simulink model "SMA_Model_Controlled"  (R2021b)
settings: Solver=FixedStepAuto  StartTime=0.0  StopTime=100  FixedStep=1e-3  RelTol=1e-3  EnableMultiTasking=on
values from neighbouring files (symbols this model uses):
  c_heat = (530.21*delta_step + 446.67*delta_ramp)    (= 513.502)    [Model_Parameters.m]
  DerivativeGain = 13.5    [Model_Parameters.m]
  diameter = 5e-4    (= 0.0005)    [Model_Parameters.m]
  Ea = (75.896*delta_step + 80.942*delta_ramp)    (= 76.9052)    [Model_Parameters.m]
  Em = (45*delta_step + 45*delta_ramp)    (= 45)    [Model_Parameters.m]
  h = (39.765*delta_step + 28.06*delta_ramp)    (= 37.424)    [Model_Parameters.m]
  Initial_Rm = 1    [Model_Parameters.m]
  Initial_temperature = (25.147*delta_step + 26.734*delta_ramp)    (= 25.4644)    [Model_Parameters.m]
  IntegralGain = 0.275    [Model_Parameters.m]
  k1 = 0.0149669    [Model_Parameters.m]
  k2 = 0.001293    [Model_Parameters.m]
  L_init = 1.0    (= 1)    [Model_Parameters.m]
  lo = 1-0.0137    (= 0.9863)    [Model_Parameters.m]
  mu_minus = (52.26*delta_step + 52.208*delta_ramp)    (= 52.2496)    [Model_Parameters.m]
  mu_plus = (56.727*delta_step + 56.131*delta_ramp)    (= 56.6078)    [Model_Parameters.m]
  mVP = 0.020563    [Model_Parameters.m]
  PropotionalGain = 950    [Model_Parameters.m]
  qVP = -0.003866    [Model_Parameters.m]
  R = (3.1232*delta_step + 2.1253*delta_ramp)    (= 2.92362)    [Model_Parameters.m]
  rho = (5392.4*delta_step + 4835.5*delta_ramp)    (= 5281.02)    [Model_Parameters.m]
  sigma_minus = (8.711*delta_step + 8.5833*delta_ramp)    (= 8.68546)    [Model_Parameters.m]
  sigma_plus = (7.9951*delta_step + 8*delta_ramp)    (= 7.99608)    [Model_Parameters.m]
  Slider_Friction = (2.6643*delta_step + 0.84475*delta_ramp)    (= 2.30039)    [Model_Parameters.m]
  Slider_Mass = (0.020002*delta_step + 0.020016*delta_ramp)    (= 0.0200048)    [Model_Parameters.m]
  SupplyVoltage = (25.001*delta_step + 25.988*delta_ramp)    (= 25.1984)    [Model_Parameters.m]
  T_amb = (26.221*delta_step + 26.843*delta_ramp)    (= 26.3454)    [Model_Parameters.m]
libraries: fl_lib x7, simulink x5, ec_arm_cortex_a_lib x4, nesl_utility x4, dspsrcs4 x1
settings Model: ExtModeTrigDuration=1000000  Creator=barag  LastModifiedBy=barag
settings SolverCC: ZeroCrossAlgorithm=Adaptive  PositivePriorityOrder=on  AutoInsertRateTranBlk=on
settings OptimizationCC: EnhancedBackFolding=on  PassReuseOutputArgsAs=Individual arguments  ZeroExternalMemoryAtStartup=off  ZeroInternalMemoryAtStartup=off  MaxStackSize=64  OptimizeBlockOrder=speed  DifferentSizesBufferReuse=on  OptimizationCustomize=off  EfficientTunableParamExpr=on
settings DebuggingCC: MaskedZcDiagnostic=none  IgnoredZcDiagnostic=none  ParameterTunabilityLossMsg=error
settings HardwareCC: ProdBitPerPointer=32  ProdBitPerSizeT=32  ProdBitPerPtrDiffT=32  ProdLargestAtomicInteger=Long  ProdLargestAtomicFloat=Double  ProdWordSize=32  ProdHWDeviceType=ARM Compatible->ARM Cortex
settings SFSimCC: MATLABDynamicMemAlloc=off
settings RTWCC: Description=Embedded Coder  SystemTargetFile=ert.tlc  HardwareBoard=BeagleBone Black  TLCOptions="-aInlineSetEventsForThisBaseRateFcn=TLC_FALSE -aSuppressMultiTaskScheduler=TLC_FALSE  -aRateBasedStepFcn=0"  TemplateMakefile=ert_default_tmf  Toolchain=Linaro Toolchain v4.8
settings CodeAppCC: ForceParamTrailComments=on  IgnoreCustomStorageClasses=off  OperatorAnnotations=on  SimulinkDataObjDesc=on  SFDataObjDesc=on  InsertBlockDesc=on
settings ERTTargetCC: SupportContinuousTime=on

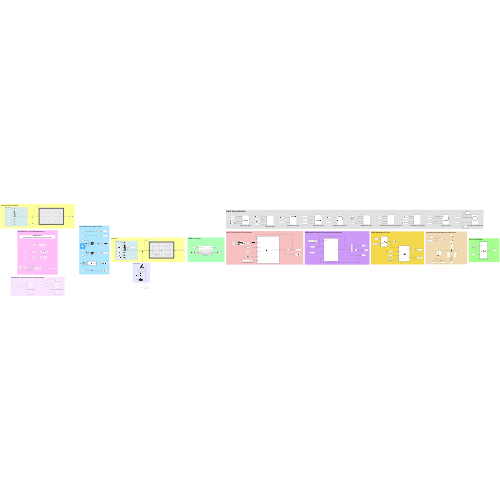
[thumbnail: Simulink's stored preview of the top-level diagram]
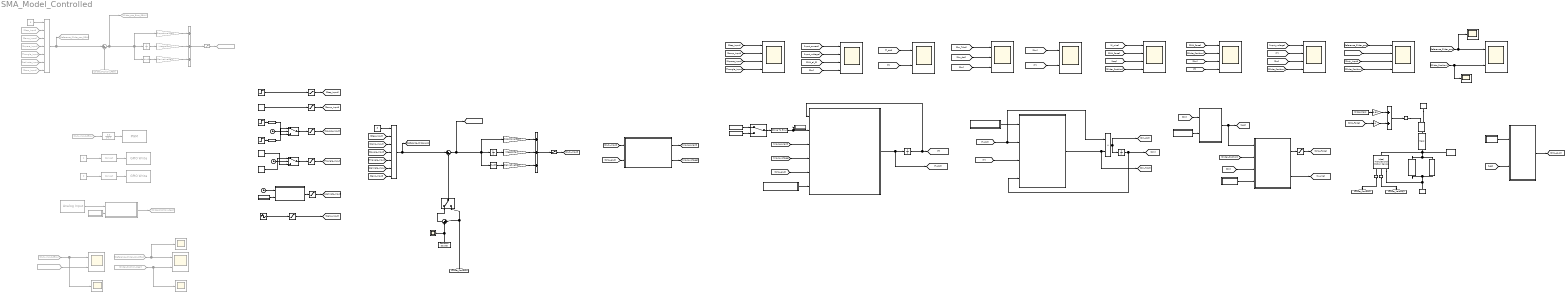
== system SMA_Model_Controlled ==
  note: WorkBench Performance Testing Scope
  note: PID
  note: Workbanch In-Out Management
  note: PWM Converter
  note: Control Real System
  note: Workbanch 15
      | max delta position 1.68cm (from 1.005V to 0.188V)
  note: Electrical Model
  note: SMA Mechanical Force
  note: Setup Mechanical Model (Simscape)
  note: Data Visualization
  note: Martensite Fraction-Temperature Hysteresis
  note: Heat Transfer and Temperature
  note: Constant Duty Cycle Inputs
  note: Input Selector
  note: Sensor Noise
  note: PID
  note: Control
  note: Input Selector
  Add : Sum
  Add1 : Sum  Commented=on  Inputs=+++
  Add2 : Sum  Inputs=+++
  Analog Input1 : ec_arm_cortex_a_lib/Analog Input  Commented=on  board=BeagleBone Black  pin=P9_33  sampleTime=0.01  blockPlatform=BeagleBone
      settings: SourceProductBaseCode=ECCORTEXA
  Constant : Constant  Commented=on  Value=6
  Constant1 : Constant  Value=3
  Constant3 : Constant  Value=Slider_Mass
  Constant4 : Constant  Commented=on  Value=0
  Control Signals : Scope  Commented=on  NumInputPorts=2
  Control scope : Scope  NumInputPorts=4
  Controlled_Displacement : Scope  NumInputPorts=2
  Data Type Conversion1 : DataTypeConversion  Commented=on
  Data Type Conversion2 : DataTypeConversion  Commented=on
  Derivative : Derivative  Commented=on
  Derivative1 : Derivative
  Discrete Transfer Fcn1 : DiscreteTransferFcn  Commented=on  Numerator=[0.3]  Denominator=[1 -0.7]
  Display : Display
  Duty_Input_Type : Scope  NumInputPorts=4
  Electrical scope : Scope  NumInputPorts=4
  From18 : From  Commented=on  GotoTag=Step_Input
  From23 : From  Commented=on  GotoTag=Ramp_Input
  From24 : From  Commented=on  GotoTag=Square_Input
  From28 : From  Commented=on  GotoTag=Triangle_Input
  From33 : From  Commented=on  GotoTag=Duty_Input_REAL
  From42 : From  Commented=on  GotoTag=Scalinata_Input
  From51 : From  Commented=on  GotoTag=Seno_Input
  From52 : From  Commented=on  GotoTag=Reference_Slider_pos_REAL
  From53 : From  Commented=on  GotoTag=Slider_Position_Real
  From54 : From  Commented=on  GotoTag=Duty_Input_REAL
  From57 : From  Commented=on  GotoTag=Slider_pos_Error_REAL
  From58 : From  Commented=on  GotoTag=Slider_Position_Real
  GPIO Write - INA : ec_arm_cortex_a_lib/GPIO Write  Commented=on  board=BeagleBone Black  gpio=P9_11  direction=Output  blockPlatform=BeagleBone
      settings: SourceProductBaseCode=ECCORTEXA
  GPIO Write - INB : ec_arm_cortex_a_lib/GPIO Write  Commented=on  board=BeagleBone Black  gpio=P9_13  direction=Output  blockPlatform=BeagleBone
      settings: SourceProductBaseCode=ECCORTEXA
  Gain : Gain  Gain=-1
  Gain1 : Gain  Commented=on  Gain=PropotionalGain
  Gain2 : Gain  Commented=on  Gain=IntegralGain
  Gain3 : Gain  Commented=on  Gain=DerivativeGain
  Gain4 : Gain  Gain=PropotionalGain
  Gain5 : Gain  Gain=IntegralGain
  Gain6 : Gain  Gain=DerivativeGain
  Goto11 : Goto  Commented=on  GotoTag=Slider_Position_Real
  Goto22 : Goto  Commented=on  GotoTag=Duty_Input_REAL
  Goto5 : Goto  Commented=on  GotoTag=Reference_Slider_pos_REAL
  Goto7 : Goto  Commented=on  GotoTag=Slider_pos_Error_REAL
  Gravity1 : Gain  Gain=9.81
  Hysteresis Parameters : Subsystem
  Hysteresis scope : Scope  NumInputPorts=3
  Ideal Force Source : fl_lib/Mechanical/Mechanical Sources/Ideal Force Source
  Ideal Translational Motion Sensor : fl_lib/Mechanical/Mechanical Sensors/Ideal Translational Motion Sensor  offset=0 m
  Input Output Comparison : Scope  NumInputPorts=4
  Input_DutyCycle_SAVING : Scope  Commented=on
  Integrator : Integrator  InitialCondition=Initial_temperature
  Integrator1 : Integrator  InitialCondition=Initial_Rm
  Integrator2 : Integrator  Commented=on
  Integrator3 : Integrator
  Leq(Rm) : MATLAB Function  TreatAsAtomicUnit=on
  MATLAB Function : MATLAB Function  TreatAsAtomicUnit=on
  MATLAB Function2 : MATLAB Function  TreatAsAtomicUnit=on
  Manual Switch : ManualSwitch
  Manual Switch3 : ManualSwitch
  Mass : fl_lib/Mechanical/Translational Elements/Mass  mass=Slider_Mass kg  num_ports=foundation.enum.numPorts2.two  v_specify=off  v_priority=High  v=0 m/s  v_nominal_specify=off  v_nominal_unit=m/s  v_nominal_value=1  f_specify=off  f_priority=None  f=0 N  f_nominal_specify=off  f_nominal_unit=N  f_nominal_value=1
      settings: InternalSimscapePortConfiguration="{\"Bottom\":[],\"Left\":[{\"id\":\"M\",\"label\":\"\",\"type\":\"foundation.mechanical.translational.translational\"}],\"Right\":[{\"id\":\"N\",\"label\":\"\",\"type\":\"foundation.mechanical.translational.translational\"}],\"Top\":[]}"
  Mechanical Translational Reference : fl_lib/Mechanical/Translational Elements/Mechanical Translational Reference
  Mechanical Translational Reference1 : fl_lib/Mechanical/Translational Elements/Mechanical Translational Reference
  Mechanical Temperature Hysteresis : Scope  NumInputPorts=4
  Mechanical scope : Scope  NumInputPorts=4
  Multiport Switch : MultiPortSwitch  Commented=on  Inputs=6
  Multiport Switch1 : MultiPortSwitch  Inputs=6
  ON : Constant  Commented=on
  PS-Simulink Converter : nesl_utility/PS-Simulink Converter  PhysicalDomain=network_engine_domain  SubClassName=ps_output  LeftPortType=input  RightPortType=output  PseudoPeriodic=off  Frequencies=[]  Unit=inherit  AffineConversion=off
      settings: SourceProductBaseCode=PW,SS
  PS-Simulink Converter1 : nesl_utility/PS-Simulink Converter  PhysicalDomain=network_engine_domain  SubClassName=ps_output  LeftPortType=input  RightPortType=output  PseudoPeriodic=off  Frequencies=[]  Unit=inherit  AffineConversion=off
      settings: SourceProductBaseCode=PW,SS
  PWM1 : ec_arm_cortex_a_lib/PWM  Commented=on  board=BeagleBone Black  pin=P9_21  frequency=20000  polarity=Positive  blockPlatform=BeagleBone
      settings: SourceProductBaseCode=ECCORTEXA
  PWM_Converter : Subsystem
  Parameters : Subsystem
  Parameters1 : Subsystem
  ParametesVP : Subsystem  Commented=on
  Product : Product
  Ramp1 : simulink/Sources/Ramp  slope=((L_init-lo)*0.8)/30  start=10  InitialOutput=0
  Ramp3 : simulink/Sources/Ramp  slope=((L_init-lo)*0.4)/15  start=5  InitialOutput=0
  Ramp4 : simulink/Sources/Ramp  slope=-((L_init-lo)*0.4)/15  start=40  InitialOutput=(L_init-lo)
  Ramp_Time_Trigger : Clock
  Random Source1 : dspsrcs4/Random Source  SrcType=Uniform  NormMethod=Ziggurat  CltLength=12  MinVal=-0.00005  MaxVal=0.00005  MeanVal=0  VarVal=0.00000025  RepMode=Not repeatable  rawSeed=1  IsInherit=off  SampMode=Continuous  SampTime=1  SampFrame=1  DataType=Single  OutComplex=Real  OutputFrames=off
  SMA_Electric_Resistance_LinearModel : MATLAB Function  TreatAsAtomicUnit=on
  SMA_Wire_Force1 : MATLAB Function  TreatAsAtomicUnit=on
  Saturation{,1,4,6,8} (5 alike) : Saturate  UpperLimit=(L_init-lo)  LowerLimit=0
  Saturation2 : Saturate  UpperLimit=1000  LowerLimit=-260.27
  Saturation3 : Saturate  Commented=on  UpperLimit=0.25  LowerLimit=0
  Saturation5 : Saturate  UpperLimit=(L_init-lo)*0.8  LowerLimit=0
  Saturation7 : Saturate  UpperLimit=0.25  LowerLimit=0
  Scalinata Signal : MATLAB Function  TreatAsAtomicUnit=on
  Scalinata_Time_Trigger1 : Clock
  Scope1 : Scope
  SensorPosition_SAVING : Scope  Commented=on
  SensorPosition_SAVING1 : Scope  Commented=on
  SensorPosition_SAVING2 : Scope
  SensorPosition_SAVING3 : Scope
  Simulink-PS Converter : nesl_utility/Simulink-PS Converter  PhysicalDomain=network_engine_domain  SubClassName=ps_input  LeftPortType=input  RightPortType=output  PseudoPeriodic=off  Frequencies=[]  NoiseDistribution=none  NoiseParameters=[]  Unit=1  AffineConversion=off  FilteringAndDerivatives=provide  SimscapeFilterOrder=1  InputFilterTimeConstant=0.001  UdotUserProvided=0
      settings: SourceProductBaseCode=PW,SS
  Sine Wave : Sin  Amplitude=(L_init-lo)*0.5*0.8  Bias=(L_init-lo)*0.5*0.8  Frequency=1/9  Phase=(3/2)*pi  SampleTime=0
  Slider Gain : simulink/Math Operations/Slider Gain  gain=1  low=0.8  high=1
  Slider Gain1 : simulink/Math Operations/Slider Gain  gain=1  low=0.8  high=1
  Solver Configuration : nesl_utility/Solver Configuration  PhysicalDomain=network_engine_domain  SubClassName=solver  LeftPortType=input  RightPortType=generic  Tones=[]  Harmonics=[]  SimulateNoise=off  Profile=off  UseLocalSampling=off  EnableSwitchedLinearOptims=on  FrequencyDomain=off  UseCCode=off  RelTol=0.001  AbsTol=1e-06  MinStep=1e-09  ToWorkspace=off  RevertToSquareIcSolve=off  NumHomotopyIterations=100  PhasorMode=off  PhasorModeNumHarmonics=1  DoDC=on  ResidualTolerance=1e-09  UseLocalSolver=off  LocalSolverChoice=NE_BACKWARD_EULER_ADVANCER  LocalSolverSampleTime=0.001  DoFixedCost=off  MaxNonlinIter=3  MaxModeIter=2  ComputeImpulses=off  ImpulseIterations=2  LinearAlgebra=auto  EquationFormulation=NE_TIME_EF  DelaysMemoryBudget=1024  AutomaticFiltering=on  FilteringTimeConstant=0.001  PartitionStorageMethod=AS_NEEDED  PartitionMemoryBudget=1024  PartitionMethod=ROBUST
      settings: SourceProductBaseCode=PW,SS
  Step1 : Step  Time=10  After=((L_init-lo)*0.8)  SampleTime=0
  Step3 : Step  Time=30  Before=((L_init-lo))  After=0  SampleTime=0
  Step4 : Step  Time=10  After=((L_init-lo))  SampleTime=0
  Step_Time_Trigger : Clock
  String Constant : StringConstant  String="\"voltage\""
  String Constant1 : StringConstant  String="\"current\""
  String to Enum : StringToEnum  OutDataTypeStr=Enum: ElectricalInputType
  Subsystem1 : Subsystem
  Sum : Sum  Commented=on  Inputs=|+-
  Sum2 : Sum  Inputs=|+-
  Sum3 : Sum  Inputs=|++
  Switch1 : Switch  Criteria=u2 > Threshold  Threshold=30
  Switch2 : Switch  Criteria=u2 > Threshold  Threshold=40
  Temperature Hysteresis : Scope  NumInputPorts=2
  Temperature scope : Scope  NumInputPorts=2
  Tracking Performance : Scope  Commented=on  NumInputPorts=2
  Translational Damper : fl_lib/Mechanical/Translational Elements/Translational Damper  D=Slider_Friction N/(m/s)  v_specify=off  v_priority=None  v=0 m/s  v_nominal_specify=off  v_nominal_unit=m/s  v_nominal_value=1  f_specify=off  f_priority=None  f=0 N  f_nominal_specify=off  f_nominal_unit=N  f_nominal_value=1
  Translational Spring : fl_lib/Mechanical/Translational Elements/Translational Spring  spr_rate=Spring_Stiff N/m  v_specify=off  v_priority=None  v=0 m/s  v_nominal_specify=off  v_nominal_unit=m/s  v_nominal_value=1  f_specify=off  f_priority=High  f=9 N  f_nominal_specify=off  f_nominal_unit=N  f_nominal_value=1  x_specify=off  x_priority=High  x=0 m  x_nominal_specify=off  x_nominal_unit=m  x_nominal_value=1
  Volt_to_Position : MATLAB Function  Commented=on  TreatAsAtomicUnit=on
  convective heat transfer parameters : Subsystem
  parameters1 : Subsystem
  wires:
  MATLAB Function/1(Temperature_dot) -> Integrator/1, [T_dot]  "T_dot"
  Integrator/1 -> MATLAB Function/1(T), [T]  "T"
  convective heat transfer parameters/1(Parameters) -> MATLAB Function/6(Parameters)
  Hysteresis Parameters/1(Parameters) -> MATLAB Function2/1(Parameters)
  [T_dot] -> MATLAB Function2/2(T_dot), Product/1  "T_dot"
  MATLAB Function2/1(Rm_Tdot) -> Product/2, [Rm_Tdot]  "Rm_dot"
  [T_dot] -> Temperature scope/1  "T_dot"
  [T] -> Temperature scope/2  "T"
  [Rm_Tdot] -> Hysteresis scope/1  "Rm_Tdot"
  [Rm_dot] -> Hysteresis scope/2  "Rm_dot"
  [Rm] -> Hysteresis scope/3  "Rm"
  [T] -> MATLAB Function2/3(T)
  [SMA_el_R] -> MATLAB Function/5(SMA_el_R)
  Product/1 -> [Rm_dot], Integrator1/1
  SMA_Electric_Resistance_LinearModel/1(SMA_R) -> [SMA_el_R]
  [Rm] -> Electrical scope/4  "Rm"
  [SMA_el_R] -> Electrical scope/3  "Ele_Resistance"
  [input_current] -> Electrical scope/1  "Input Current"
  Parameters1/1(Parameters) -> SMA_Electric_Resistance_LinearModel/1(Parameters)
  [Leq] -> SMA_Electric_Resistance_LinearModel/2(Leq)
  PWM_Converter/2(SMA_Voltage) -> [input_voltage]
  [input_voltage] -> Electrical scope/2  "Input Voltage"
  ON/1 -> Data Type Conversion1/1
  Data Type Conversion2/1 -> GPIO Write - INB/1
  Data Type Conversion1/1 -> GPIO Write - INA/1
  Constant4/1 -> Data Type Conversion2/1
  [SMA_el_R] -> PWM_Converter/2(SMA_Resistance)
  ParametesVP/1(Parameters) -> Volt_to_Position/2(Parameters)
  Gain/1 -> Add/2
  [SMA_Force] -> Gain/1
  PS-Simulink Converter/1 -> [Slider_Velocity]  "Velocity"
  Add1/1 -> Saturation3/1
  Volt_to_Position/1(SensorPosition) -> Goto11/1
  SMA_Wire_Force1/1(SMA_Force) -> Saturation2/1
  Leq(Rm)/1(Leq) -> [Leq], SMA_Wire_Force1/1(Leq)
  SMA_Wire_Force1/2(K_wire) -> [K_wire]
  [Rm] -> SMA_Wire_Force1/3(Rm)
  parameters1/1(Parameters) -> SMA_Wire_Force1/4(Parameters)
  [Rm] -> Leq(Rm)/1(Rm)
  Subsystem1/1(Parameters) -> Leq(Rm)/2(Parameters)
  [SMA_Force] -> Mechanical scope/2  "SMA_force"
  [K_wire] -> Mechanical scope/1  "K_wire"
  [Leq] -> Mechanical scope/3  "Leq"
  [Slider_Position] -> Mechanical scope/4  "Displacement"
  Add/1 -> Simulink-PS Converter/1
  Constant3/1 -> Gravity1/1
  Gravity1/1 -> Add/1
  Discrete Transfer Fcn1/1 -> PWM1/1
  [input_voltage] -> MATLAB Function/4(Input_Voltage)
  PWM_Converter/1(SMA_Current) -> [input_current]
  [input_current] -> MATLAB Function/3(Input_Current)
  Manual Switch/1 -> String to Enum/1
  String Constant/1 -> Manual Switch/1
  String Constant1/1 -> Manual Switch/2
  [Step_Input] -> Duty_Input_Type/1  "Duty_Step_input"
  [Ramp_Input] -> Duty_Input_Type/2  "Duty_Ramp_input"
  [Square_Input] -> Duty_Input_Type/3  "Duty_Square_input"
  [Triangle_Input] -> Duty_Input_Type/4  "Duty_Triangle_input"
  String to Enum/1 -> MATLAB Function/2(Electric_Input), Display/1
  [Rm] -> Temperature Hysteresis/1  "Rm"
  [T] -> Temperature Hysteresis/2  "Temperature"
  [Rm] -> Mechanical Temperature Hysteresis/3  "Rm"
  [Slider_Position] -> Mechanical Temperature Hysteresis/2  "Displacement"
  [SMA_Force] -> Mechanical Temperature Hysteresis/1  "SMA_force"
  [T] -> Mechanical Temperature Hysteresis/4  "Temperature"
  [input_voltage] -> Input Output Comparison/1  "Input Voltage"
  [Rm] -> Input Output Comparison/3  "Rm"
  [Slider_Position] -> Input Output Comparison/4  "Displacement"
  [T] -> Input Output Comparison/2  "Temperature"
  Integrator1/1 -> [Rm], MATLAB Function2/4(Rm)
  Integrator2/1 -> Gain2/1
  Sum/1 -> Integrator2/1, Derivative/1, Gain1/1, Goto7/1  "Slider_Position_Error"
  Gain1/1 -> Add1/1
  Gain2/1 -> Add1/2
  [Duty_Input] -> PWM_Converter/1(Reference PWM Voltage)
  From58/1 -> Sum/2
  Ramp3/1 -> Switch2/3  "Increment_Ramp"
  Step4/1 -> Slider Gain1/1  "Upper_step"
  Ramp_Time_Trigger/1 -> Switch2/2
  From24/1 -> Multiport Switch/4
  From28/1 -> Multiport Switch/5
  Step_Time_Trigger/1 -> Switch1/2
  From23/1 -> Multiport Switch/3
  Switch1/1 -> Saturation4/1
  From18/1 -> Multiport Switch/2
  Saturation1/1 -> [Ramp_Input]
  Saturation4/1 -> [Square_Input]
  Saturation5/1 -> [Triangle_Input]
  Step3/1 -> Slider Gain/1  "Lower_Step"
  Ramp1/1 -> Saturation1/1  "Ramp_Input"
  Constant/1 -> Multiport Switch/1
  Switch2/1 -> Saturation5/1
  Step1/1 -> Saturation/1  "Step_Input"
  Saturation/1 -> [Step_Input]
  Ramp4/1 -> Switch2/1  "Decrement_ramp"
  [Reference_Slider_pos] -> Control scope/1  "Reference Displacement"
  [Slider_pos_Error] -> Control scope/2  "Displacement Error"
  [Duty_Input] -> Control scope/3  "Duty Cycle"
  [Slider_Position] -> Control scope/4  "Displacement"
  Saturation3/1 -> Goto22/1
  [Reference_Slider_pos] -> SensorPosition_SAVING3/1, Controlled_Displacement/1  "Reference Displacement"
  [Slider_Position] -> SensorPosition_SAVING2/1, Controlled_Displacement/2  "Model_Displacement"
  PS-Simulink Converter1/1 -> [Slider_Position]  "Position"
  Derivative/1 -> Gain3/1
  Gain3/1 -> Add1/3
  Scalinata Signal/1(Out_Signal) -> Saturation6/1
  Scalinata_Time_Trigger1/1 -> Scalinata Signal/1(time)
  Parameters/1(Out1) -> Scalinata Signal/2(Parameters)
  Saturation6/1 -> [Scalinata_Input]
  Sine Wave/1 -> Saturation8/1
  From42/1 -> Multiport Switch/6
  From51/1 -> Multiport Switch/7
  Saturation8/1 -> [Seno_Input]
  From52/1 -> SensorPosition_SAVING1/1, Tracking Performance/1  "Reference_Position"
  From53/1 -> SensorPosition_SAVING/1, Tracking Performance/2  "Measured_Position"
  From54/1 -> Input_DutyCycle_SAVING/1, Control Signals/1  "Duty_Input"
  From57/1 -> Control Signals/2  "Tracking_Error"
  [Seno_Input] -> Multiport Switch1/7
  [Scalinata_Input] -> Multiport Switch1/6
  Gain6/1 -> Add2/3
  Derivative1/1 -> Gain6/1
  Random Source1/1 -> Scope1/1, Sum3/2
  [Slider_Position] -> Sum3/1, Manual Switch3/2
  Sum3/1 -> Manual Switch3/1
  Saturation7/1 -> [Duty_Input]
  Constant1/1 -> Multiport Switch1/1
  [Step_Input] -> Multiport Switch1/2
  [Ramp_Input] -> Multiport Switch1/3
  [Triangle_Input] -> Multiport Switch1/5
  [Square_Input] -> Multiport Switch1/4
  Multiport Switch1/1 -> Sum2/1, [Reference_Slider_pos]
  Manual Switch3/1 -> Sum2/2
  Gain5/1 -> Add2/2
  Gain4/1 -> Add2/1
  Sum2/1 -> [Slider_pos_Error], Gain4/1, Derivative1/1, Integrator3/1  "Slider_Position_Error"
  Integrator3/1 -> Gain5/1
  Add2/1 -> Saturation7/1
  [Slider_Position] -> SMA_Wire_Force1/2(Delta_L)
  From33/1 -> Discrete Transfer Fcn1/1
  Analog Input1/1 -> Volt_to_Position/1(SensorVolt)
  Multiport Switch/1 -> Sum/1, Goto5/1
  Saturation2/1 -> [SMA_Force]
  Slider Gain/1 -> Switch1/1
  Slider Gain1/1 -> Switch1/3
  connections:
  Solver Configuration/RConn1 -- Translational Damper/LConn1 -- Translational Spring/LConn1 -- Mass/LConn1 -- Ideal Translational Motion Sensor/LConn1
  Mechanical Translational Reference/LConn1 -- Translational Damper/RConn1 -- Translational Spring/RConn1 -- Ideal Translational Motion Sensor/RConn1
  Mechanical Translational Reference1/LConn1 -- Ideal Force Source/RConn2
  PS-Simulink Converter/LConn1 -- Ideal Translational Motion Sensor/RConn2
  PS-Simulink Converter1/LConn1 -- Ideal Translational Motion Sensor/RConn3
  Simulink-PS Converter/RConn1 -- Ideal Force Source/RConn1
  Mass/RConn1 -- Ideal Force Source/LConn1

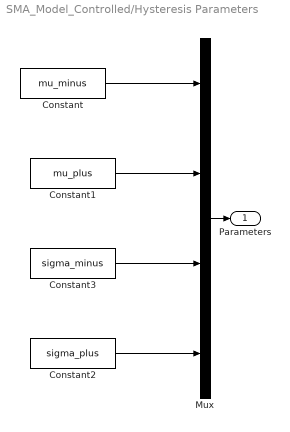
== system SMA_Model_Controlled/Hysteresis Parameters ==
  Constant : Constant  Value=mu_minus
  Constant1 : Constant  Value=mu_plus
  Constant2 : Constant  Value=sigma_plus
  Constant3 : Constant  Value=sigma_minus
  Mux : Mux
  Parameters : Outport
  wires:
  Mux/1 -> Parameters/1
  Constant2/1 -> Mux/4
  Constant/1 -> Mux/1
  Constant1/1 -> Mux/2
  Constant3/1 -> Mux/3

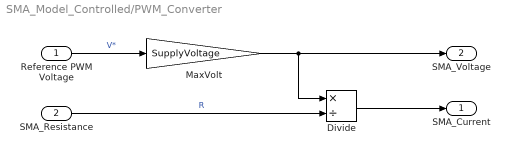
== system SMA_Model_Controlled/PWM_Converter ==
  Reference PWM Voltage : Inport
  SMA_Resistance : Inport  Port=2
  Divide : Product  Inputs=*/
  MaxVolt : Gain  Gain=SupplyVoltage
  SMA_Current : Outport
  SMA_Voltage : Outport  Port=2
  wires:
  Reference PWM Voltage/1 -> MaxVolt/1  "V*"
  MaxVolt/1 -> Divide/1, SMA_Voltage/1
  Divide/1 -> SMA_Current/1
  SMA_Resistance/1 -> Divide/2  "R"

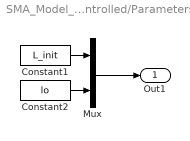
== system SMA_Model_Controlled/Parameters ==
  Constant1 : Constant  Value=L_init
  Constant2 : Constant  Value=lo
  Mux : Mux  Inputs=2
  Out1 : Outport
  wires:
  Constant2/1 -> Mux/2
  Mux/1 -> Out1/1
  Constant1/1 -> Mux/1

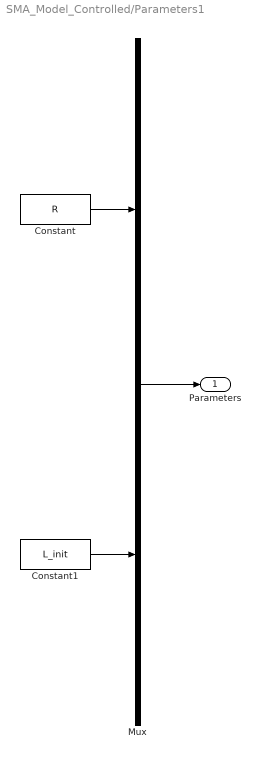
== system SMA_Model_Controlled/Parameters1 ==
  Constant : Constant  Value=R
  Constant1 : Constant  Value=L_init
  Mux : Mux  Inputs=2
  Parameters : Outport
  wires:
  Mux/1 -> Parameters/1
  Constant/1 -> Mux/1
  Constant1/1 -> Mux/2

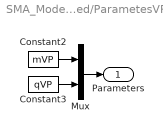
== system SMA_Model_Controlled/ParametesVP ==
  Constant2 : Constant  Value=mVP
  Constant3 : Constant  Value=qVP
  Mux : Mux  Inputs=2
  Parameters : Outport
  wires:
  Constant2/1 -> Mux/1
  Constant3/1 -> Mux/2
  Mux/1 -> Parameters/1

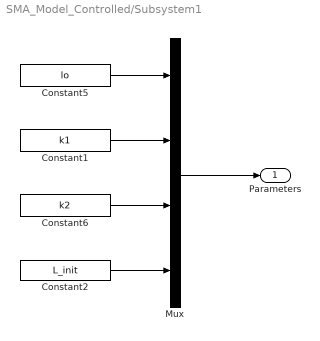
== system SMA_Model_Controlled/Subsystem1 ==
  Constant1 : Constant  Value=k1
  Constant2 : Constant  Value=L_init
  Constant5 : Constant  Value=lo
  Constant6 : Constant  Value=k2
  Mux : Mux
  Parameters : Outport
  wires:
  Constant6/1 -> Mux/3
  Constant1/1 -> Mux/2
  Constant5/1 -> Mux/1
  Mux/1 -> Parameters/1
  Constant2/1 -> Mux/4

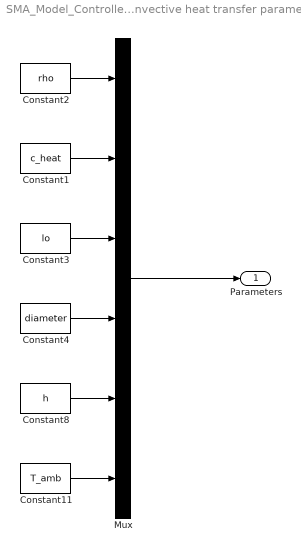
== system SMA_Model_Controlled/convective heat transfer parameters ==
  Constant1 : Constant  Value=c_heat
  Constant11 : Constant  Value=T_amb
  Constant2 : Constant  Value=rho
  Constant3 : Constant  Value=lo
  Constant4 : Constant  Value=diameter
  Constant8 : Constant  Value=h
  Mux : Mux  Inputs=6
  Parameters : Outport
  wires:
  Constant8/1 -> Mux/5
  Constant2/1 -> Mux/1
  Constant1/1 -> Mux/2
  Constant3/1 -> Mux/3
  Constant4/1 -> Mux/4
  Mux/1 -> Parameters/1
  Constant11/1 -> Mux/6

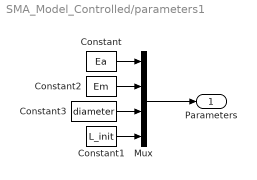
== system SMA_Model_Controlled/parameters1 ==
  Constant : Constant  Value=Ea
  Constant1 : Constant  Value=L_init
  Constant2 : Constant  Value=Em
  Constant3 : Constant  Value=diameter
  Mux : Mux
  Parameters : Outport
  wires:
  Constant1/1 -> Mux/4
  Mux/1 -> Parameters/1
  Constant/1 -> Mux/1
  Constant3/1 -> Mux/3
  Constant2/1 -> Mux/2

== matlab function SMA_Model_Controlled/SMA_Wire_Force1 ==
  data: Leq input; Delta_L input; SMA_Force output; Rm input; Parameters input; K_wire output
function [SMA_Force, K_wire]= SMA_force(Leq, Delta_L, Rm, Parameters)
% Parameters
Ea =     Parameters(1)*1e9; % from [GPa] to [Pa]
Em =     Parameters(2)*1e9; % from [GPa] to [Pa]
do =     Parameters(3);
L_init = Parameters(4);

% Wire sectional area
A_wire = (do/2)^2 * pi;

% Wire Stiffness Coefficient
% K_wire = (Rm*Em + (1-Rm)*Ea)* A_wire;
 K_wire = (Rm*Em + (1-Rm)*Ea)* A_wire/(L_init-Leq);

%L_in = (Rm*L_init + (1-Rm)*L_init*0.986);

% deformation
% epsilon = Delta_L;
% epsilon_init = L_init;
% 
% Normalized_displacement = epsilon + epsilon_init;


% Force generated by the SMA wire 
SMA_Force = K_wire *(Delta_L - Leq);

== matlab function SMA_Model_Controlled/MATLAB Function ==
  data: T input; Electric_Input input; Input_Current input; Input_Voltage input; SMA_el_R input; Parameters input; Temperature_dot output
function Temperature_dot = Convective_Heat_Transfer_Equation( T, Electric_Input, Input_Current, Input_Voltage, SMA_el_R, Parameters)
% Parameters Estraztion
rho =    Parameters(1); % mass density of SMA wire[kgm-3]
c_heat = Parameters(2); % specific heat of SMA wire [Jkg-1C-1]
lo =     Parameters(3); % undeformed SMA wire length in 100% A state [m]
do =     Parameters(4); % cross-sectional diameter of undeformed SMA wire [m]
h =      Parameters(5); % convection heat transfer coefficient [Wm-2C-1]
T_amb =  Parameters(6); % ambient temperature [C]

% Equation Terms Definitions:
Term_1 = (rho*c_heat*pi*lo*(do^2))/4;
%Term_2 = (1+(eps/2))*p1*do*Lo*h;
Term_2_simplified = pi*do*lo*h;


% Electrical Power
if Electric_Input == 0
    El_Pow_Term = (Input_Voltage^2)/SMA_el_R;

elseif Electric_Input == 1
    El_Pow_Term = SMA_el_R*(Input_Current^2);

else
    El_Pow_Term = Input_Voltage*Input_Current;
end

T_diff = T - T_amb;

% Temperature Rate of Variation :
Temperature_dot = (El_Pow_Term - Term_2_simplified*T_diff)/Term_1; %
%Simplified version with eps assumed to be small and neglectable
%Temperature_dot = (El_Pow_Term - Term_2*T_diff)/Term_1;

== matlab function SMA_Model_Controlled/MATLAB Function2 ==
  data: Parameters input; Rm_Tdot output; T_dot input; T input; Rm input
function Rm_Tdot = Hysteresis(Parameters, T_dot, T, Rm)
    % Parameter Extraction
    mu_minus =    Parameters(1);
    mu_plus =     Parameters(2);
    sigma_minus = Parameters(3);
    sigma_plus =  Parameters(4);

    ER_minus = erf((T-mu_minus)/(sigma_minus*sqrt(2)));
    ER_plus = erf((T-mu_plus)/(sigma_plus*sqrt(2)));

    H_minus = 0.5 * (1 + ER_minus);
    H_plus  = 0.5 * (1 + ER_plus);

    Exp_minus = exp(-((T-mu_minus)/(sigma_minus*sqrt(2)))^2);
    Exp_plus  = exp(-((T-mu_plus)/(sigma_plus*sqrt(2)))^2);

    Gauss_minus= (1/(sigma_minus*sqrt(2*pi)))*Exp_minus;
    Gauss_plus = (1/(sigma_plus*sqrt(2*pi)))*Exp_plus;
    
    Rm_Tdot=0;
    if T_dot >= 0
        ceff_plus = (H_minus + Rm - 1)/(H_plus - H_minus + 0.0000001);
        Rm_Tdot = ceff_plus*Gauss_plus;
    elseif T_dot < 0
        ceff_minus = (H_plus + Rm - 1)/(H_minus - H_plus +0.001);
        Rm_Tdot = ceff_minus*Gauss_minus;
    end 
%   if Rm_Tdot == 0
%       Rm_Tdot = 1e-6;
%   end
end

== matlab function SMA_Model_Controlled/Scalinata Signal ==
  data: time input; Out_Signal output; Parameters input
function Out_Signal = Scalinata(time, Parameters)

L_init = Parameters(1);
lo     = Parameters(2);

Max_disp = (L_init-lo)*0.8;

gimmy = 0;

     if time >= 10 
        gimmy = Max_disp/5;
     end
     if time >= 20
         gimmy = (Max_disp*2)/5;
     end
     if time >= 30
         gimmy = (Max_disp*3)/5;
     end
     if time >= 40
         gimmy = (Max_disp*4)/5;
     end
     if time >= 50 
         gimmy = Max_disp;
     end
     if time >= 70
         gimmy = 0;
     end

Out_Signal = gimmy;

== matlab function SMA_Model_Controlled/SMA_Electric_Resistance_LinearModel ==
  data: Parameters input; SMA_R output; Leq input
function SMA_R = SMA_Resistance(Parameters, Leq)

% Parameters Extraction
R0 = Parameters(1); % [Ohm/m] 
L_init = Parameters(2);

Lo = L_init - Leq;

%SMA Wire Electical Resistance
SMA_R = R0 * Lo;

== matlab function SMA_Model_Controlled/Volt_to_Position ==
  data: SensorVolt input; SensorPosition output; Parameters input
function SensorPosition = fcn(SensorVolt, Parameters)

m = Parameters(1);
q = Parameters(2);

SensorPosition = m*SensorVolt + q;

== matlab function SMA_Model_Controlled/Leq(Rm) ==
  data: Rm input; Leq output; Parameters input
function Leq= Equilibrium_lenght(Rm, Parameters)

% Parameters
lo     = Parameters(1);
k1     = Parameters(2);
k2     = Parameters(3);
L_init = Parameters(4);


% Wire sectional area
%A_wire = (do/2)^2 * pi;

%eps_0 = (1 - sqrt(1 - (4*k*Delta)/(A_wire*Ea)))/2;
eps_0 = 0;

eps_r = k1*Rm + k2*(Rm^2) ;

Lo = ( 1 + eps_0 + eps_r ) * lo;

Leq = L_init - Lo;
